simulink model "buck_boost_eFL"  (R2025a)
settings: Solver=ode3  StartTime=0.0  StopTime=1  FixedStep=1e-3  RelTol=1e-3  EnableMultiTasking=on
values from neighbouring files (symbols this model uses):
  C = 470*10^-6    (= 0.00047)    [projekat_2.m]
  den_NF = [1/400 1]    [projekat_2.m]
  E = 12    [projekat_2.m]
  k0 = 27*w0^2    (= 38988)    [projekat_2.m]
  k1 = 9*w0    (= 342)    [projekat_2.m]
  ki = 27*w0^3    (= 1481544)    [projekat_2.m]
  L = 15.91e-3    (= 0.01591)    [projekat_2.m]
  noise_var = (0.03*Vc)^2    (= 0.455625)    [projekat_2.m]
  num_NF = [1]    [projekat_2.m]
  R = 52    [projekat_2.m]
  sel = 1    [projekat_2.m]
  x2e = Vc    (= -22.5)    [projekat_2.m]
settings Model: Creator=Stevica  LastModifiedBy=PC
settings SolverCC: AlgebraicLoopSolver=TrustRegion
settings DataIOCC: LimitDataPoints=on  SaveFormat=Array  ReturnWorkspaceOutputs=off
settings OptimizationCC: LifeSpan=inf
settings DebuggingCC: UnderspecifiedInitializationDetection=Classic  MergeDetectMultiDrivingBlocksExec=none  SolverPrmCheckMsg=warning  UnconnectedInputMsg=warning  UnconnectedOutputMsg=warning  UnconnectedLineMsg=warning  SFUnexpectedBacktrackingDiag=warning  SFNoUnconditionalDefaultTransitionDiag=warning  SFExecutionAtInitializationDiag=none  ArithmeticOperatorsInVariantConditions=warning
settings HardwareCC: ProdBitPerPointer=32.0  ProdBitPerSizeT=32.0  ProdBitPerPtrDiffT=32.0  ProdLargestAtomicFloat=None  ProdIntDivRoundTo=Undefined  ProdEndianess=Unspecified  ProdWordSize=32.0  ProdHWDeviceType=32-bit Generic
settings ModelReferenceCC: PropagateSignalLabelsOutOfModel=off
settings SFSimCC: SimUseLocalCustomCode=off  CustomCodeUndefinedFunction=UseInterfaceOnly
settings RTWCC: RTWUseLocalCustomCode=off  GPUComputeCapability=3.5
settings CodeAppCC: StateflowObjectComments=on
settings GRTTargetCC: TargetLangStandard=C89/C90 (ANSI)
settings ConfigComp: CovMetricSettings=dw  CovSaveCumulativeToWorkspaceVar=on  CovSaveSingleToWorkspaceVar=on  CovExternalEMLEnable=off

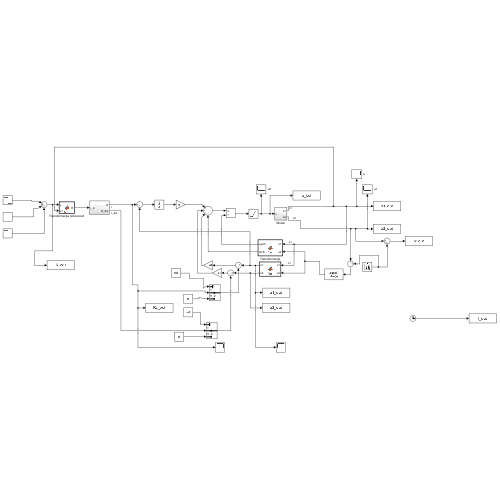
[thumbnail: Simulink's stored preview of the top-level diagram]
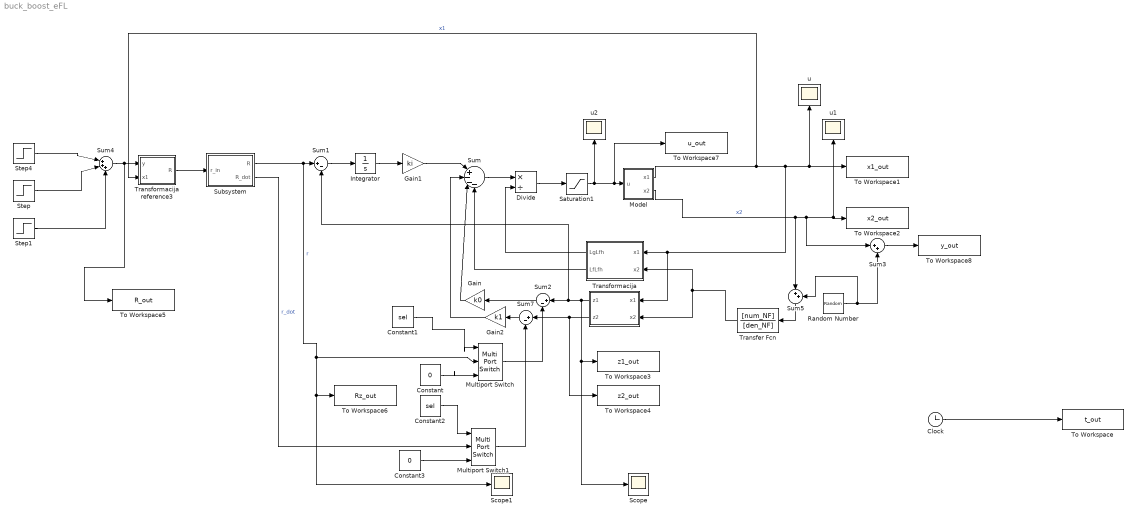
== system buck_boost_eFL ==
  " " : MATLAB Function  TreatAsAtomicUnit=on
  Clock : Clock
  Constant : Constant  Value=0
  Constant1 : Constant  Value=sel
  Constant2 : Constant  Value=sel
  Constant3 : Constant  Value=0
  Divide : Product  Inputs=*/
  Gain : Gain  Gain=k0
  Gain1 : Gain  Gain=ki
  Gain2 : Gain  Gain=k1
  Integrator : Integrator
  Model : Subsystem
  Multiport Switch : MultiPortSwitch  Inputs=2  SaturateOnIntegerOverflow=off  InputSameDT=off
  Multiport Switch1 : MultiPortSwitch  Inputs=2  SaturateOnIntegerOverflow=off  InputSameDT=off
  Random Number : RandomNumber  Variance=noise_var  SampleTime=0.001
  Saturation1 : Saturate  UpperLimit=0.9  LowerLimit=0.2
  Scope : Scope
      settings: ActiveDisplayYMinimum=-0.24329937413818187  ActiveDisplayYMaximum=0.11611023568362981  DataLoggingVariableName=ScopeData2
  Scope1 : Scope
      settings: ActiveDisplayYMinimum=-0.20338157972299231  ActiveDisplayYMaximum=0.05846526954161628  DataLoggingVariableName=ScopeData4
  Step : Step  Time=0.3  After=5  SampleTime=0
  Step1 : Step  Time=0.5  After=-5  SampleTime=0
  Step4 : Step  Time=0  After=x2e  SampleTime=0
  Subsystem : Subsystem
  Sum : Sum  Inputs=|+---
  Sum1 : Sum  Inputs=|+-
  Sum2 : Sum  Inputs=|+-
  Sum3 : Sum  Inputs=|++
  Sum4 : Sum  Inputs=|+++
  Sum5 : Sum  Inputs=|++
  Sum7 : Sum  Inputs=|+-
  To Workspace : ToWorkspace  VariableName=t_out  SampleTime=-1
  To Workspace1 : ToWorkspace  VariableName=x1_out  SampleTime=-1
  To Workspace2 : ToWorkspace  VariableName=x2_out  SampleTime=-1
  To Workspace3 : ToWorkspace  VariableName=z1_out  SampleTime=-1
  To Workspace4 : ToWorkspace  VariableName=z2_out  SaveFormat=Timeseries  SampleTime=-1
  To Workspace5 : ToWorkspace  VariableName=R_out  SampleTime=-1
  To Workspace6 : ToWorkspace  VariableName=Rz_out  SampleTime=-1
  To Workspace7 : ToWorkspace  VariableName=u_out  SampleTime=-1
  To Workspace8 : ToWorkspace  VariableName=y_out  SampleTime=-1
  Transfer Fcn : TransferFcn  Numerator=[num_NF]  Denominator=[den_NF]
  Transformacija : MATLAB Function  TreatAsAtomicUnit=on
  Transformacija reference3 : MATLAB Function  TreatAsAtomicUnit=on
  u : Scope
      settings: ActiveDisplayYMinimum=-26.055814050489122  ActiveDisplayYMaximum=-12.05466053748558
  u1 : Scope
      settings: ActiveDisplayYMinimum=-68.250155739927052  ActiveDisplayYMaximum=40.421023123891985
  u2 : Scope
      settings: ActiveDisplayYMinimum=0.059949583731811584  ActiveDisplayYMaximum=1.3029432243502124  DataLoggingVariableName=ScopeData3
  wires:
  " "/1(LgLfh) -> Divide/2
  Sum/1 -> Divide/1
  " "/2(LfLfh) -> Sum/4
  Gain1/1 -> Sum/1
  Integrator/1 -> Gain1/1
  Gain/1 -> Sum/3
  Gain2/1 -> Sum/2
  Divide/1 -> Saturation1/1
  Saturation1/1 -> To Workspace7/1, Model/1(u), u2/1
  Sum4/1 -> Transformacija reference3/1(y), To Workspace5/1
  Step/1 -> Sum4/2
  Step1/1 -> Sum4/3
  Model/1(x1) -> Transformacija reference3/2(x1), To Workspace1/1, u/1, Transformacija/1(x1), " "/1(x1)  "x1"
  Step4/1 -> Sum4/1
  Model/2(x2) -> Sum5/1, u1/1, To Workspace2/1, Sum3/1  "x2"
  Sum2/1 -> Gain/1
  Transformacija/1(z1) -> Scope/1, To Workspace3/1, Sum1/2, Sum2/1
  Clock/1 -> To Workspace/1
  Constant/1 -> Multiport Switch/3
  Multiport Switch/1 -> Sum2/2
  Constant1/1 -> Multiport Switch/1
  Random Number/1 -> Sum5/2, Sum3/2
  Sum3/1 -> To Workspace8/1
  Sum5/1 -> Transfer Fcn/1
  Transformacija reference3/1(R) -> Subsystem/1(r_in)
  Subsystem/1(R) -> Scope1/1, To Workspace6/1, Multiport Switch/2, Sum1/1  "r"
  Transformacija/2(z2) -> Sum7/1, To Workspace4/1
  Transfer Fcn/1 -> Transformacija/2(x2), " "/2(x2)
  Sum1/1 -> Integrator/1
  Sum7/1 -> Gain2/1
  Constant2/1 -> Multiport Switch1/1
  Multiport Switch1/1 -> Sum7/2
  Constant3/1 -> Multiport Switch1/3
  Subsystem/2(R_dot) -> Multiport Switch1/2  "r_dot"

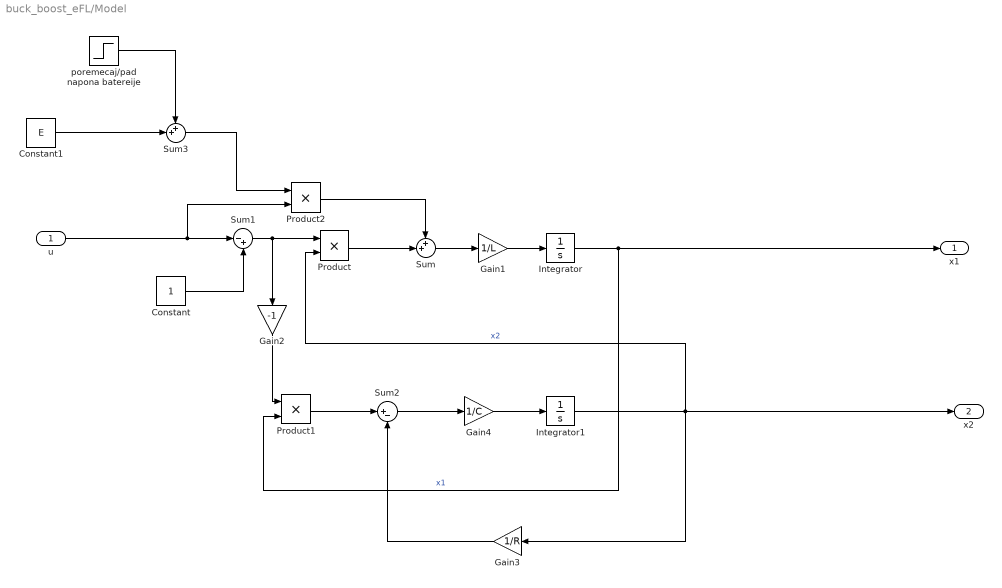
== system buck_boost_eFL/Model ==
  u : Inport
  Constant : Constant
  Constant1 : Constant  Value=E
  Gain1 : Gain  Gain=1/L
  Gain2 : Gain  Gain=-1
  Gain3 : Gain  Gain=1/R
  Gain4 : Gain  Gain=1/C
  Integrator : Integrator  LimitOutput=on  LowerSaturationLimit=0
  Integrator1 : Integrator  LimitOutput=on  UpperSaturationLimit=0
  Product : Product
  Product1 : Product
  Product2 : Product
  Sum : Sum  Inputs=++|
  Sum1 : Sum  Inputs=|-+
  Sum2 : Sum  Inputs=|+-
  Sum3 : Sum  Inputs=++|
  poremecaj/pad napona batereije : Step  Time=0.7  After=-1  SampleTime=0
  x1 : Outport
  x2 : Outport  Port=2
  wires:
  Product1/1 -> Sum2/1
  Integrator1/1 -> x2/1, Gain3/1, Product/2  "x2"
  Gain3/1 -> Sum2/2
  Constant/1 -> Sum1/2
  Sum2/1 -> Gain4/1
  Product/1 -> Sum/2
  Gain1/1 -> Integrator/1
  Sum1/1 -> Product/1, Gain2/1
  Integrator/1 -> x1/1, Product1/2  "x1"
  Product2/1 -> Sum/1
  u/1 -> Product2/2, Sum1/1
  Gain4/1 -> Integrator1/1
  Sum/1 -> Gain1/1
  Gain2/1 -> Product1/1
  Constant1/1 -> Sum3/2
  poremecaj/pad napona batereije/1 -> Sum3/1
  Sum3/1 -> Product2/1

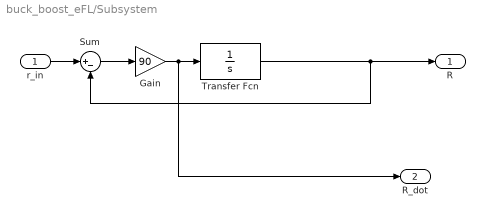
== system buck_boost_eFL/Subsystem ==
  r_in : Inport
  Gain : Gain  Gain=90
  Sum : Sum  Inputs=|+-
  Transfer Fcn : TransferFcn  Denominator=[1 0]
  R : Outport
  R_dot : Outport  Port=2
  wires:
  r_in/1 -> Sum/1
  Sum/1 -> Gain/1
  Gain/1 -> R_dot/1, Transfer Fcn/1
  Transfer Fcn/1 -> R/1, Sum/2

== matlab function buck_boost_eFL/Transformacija ==
  data: x1 input; z1 output; x2 input; z2 output
function [z1, z2] = fcn(x1, x2)

L=15.91*10^-3;
C=470*10^-6;
R=52;
E=12;

Vc=-22.5;
x2e=Vc;
x1e=1.2441;


z1 = C*x2^2 - 2*E*C*x2 + L*x1^2 - (C*x2e^2 - 2*E*C*x2e + L*x1e^2);
z2 = -2/R*x2^2 + 2*E*x1 + 2*E/R*x2;

== matlab function buck_boost_eFL/  ==
  data: x1 input; LgLfh output; x2 input; LfLfh output
function [LgLfh, LfLfh] = fcn(x1, x2)

L=15.91*10^-3;
C=470*10^-6;
R=52;
E=12;

LgLfh = -4/(R*C)*x1*x2 + 2*E/(R*C)*x1 + 2*E^2/L - 2*E/L*x2;
LfLfh = 4/(R^2*C)*x2^2 - 2*E/(R^2*C)*x2 + 2*E/L*x2 - 2*E/(R*C)*x1 +4/(R*C)*x1*x2;

== matlab function buck_boost_eFL/Transformacija reference3 ==
  data: y input; R output; x1 input
function  R= fcn(y,x1)

% y=x1e stara referenca, tj. nominalna vrednost

L=15.91*10^-3;
C=470*10^-6;
R=52;
E=12;

Vc=-22.5;
x2e=Vc;
x1e=1.2441;

gama = C*x2e^2 - 2*E*C*x2e + L*x1e^2;

R = C*y^2 - 2*E*C*y + L*(x1)^2 - gama;
